simulink model "single_sat_attitude"  (R2018a)
settings: Solver=ode1  StartTime=0.0  StopTime=10.0  FixedStep=1/100  RelTol=1e-3
undefined symbols (not defined in the file or in its folder): Earth, h_init, hdmax, hmax, IAU, init, Kd, km, Kp, NRLMSISE_time_fromJD, q_init, s, wbn_init, WGS84
libraries: aerolibtransform2 x9, aerolibutil x6, sharedtransform x4, simulink x4, aerolibcelestial x3, vrlib x3, aerolibgravity2 x2, aerolibconvert2 x2, sharedutil x2, aerolibatmos2 x1
(part 1 of 2)
settings Model: Creator=nathan  LastModifiedBy=nathan
settings SolverCC: AutoInsertRateTranBlk=on

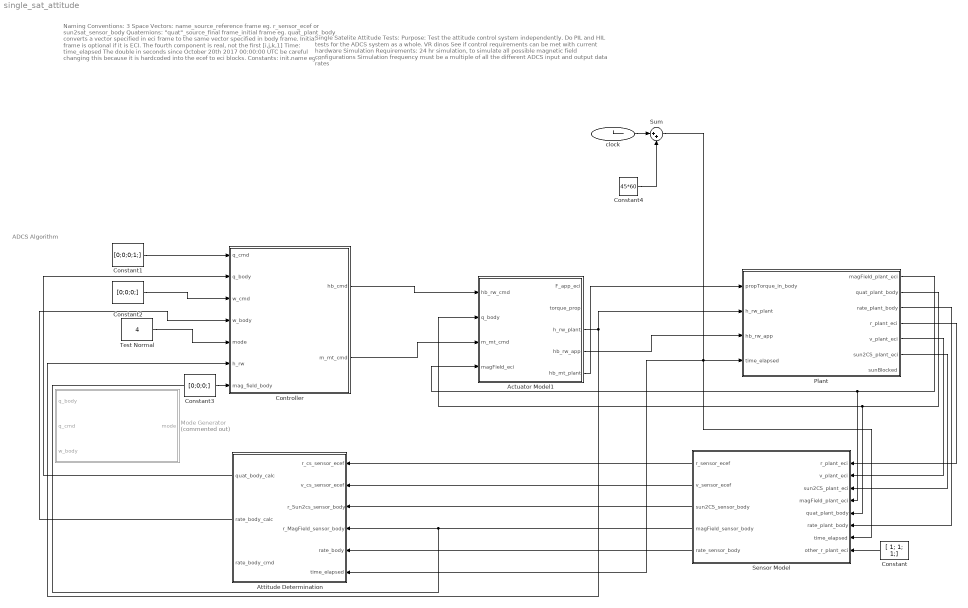
== system single_sat_attitude ==
  note: Naming Conventions:
      | 3 Space Vectors:
      | name_source_reference frame
      | eg. r_sensor_ecef or
      | sun2sat_sensor_body
      | Quaternions:
      | "quat"_source_final frame_initial frame
      | eg. quat_plant_body converts a vector specified in eci frame to the same vector specified in body frame.
      | Initial frame is optional if it is ECI.
      | The fourth component is real, not the first [i,j,k,1]
      | Time:
      | time_elapsed
      | The double in seconds since October 20th 2017 00:00:00 UTC
      | be careful changing this because it is hardcoded into the ecef to eci blocks.
      |
      | Constants:
      | init.name
      | eg. init.IMU0_MAG_RMS
      | Most constants that are not self explanitory should be stored in init. Their names must be all caps.
  note: ADCS Algorithm
  note: Single Satelite Attitude Tests:
      |
      | Purpose:
      | Test the attitude control system independently.
      | Do PIL and HIL tests for the ADCS system as a whole.
      | VR dinos
      | See if control requirements can be met with current hardware
      | Simulation Requirements:
      | 24 hr simulation, to simulate all possible magnetic field configurations
      | Simulation frequency must be a multiple of all the different ADCS input and output data rates
  Actuator Model1 : Subsystem
  Attitude Determination : Subsystem
  Constant : Constant  Value=[ 1; 1; 1;]
  Constant1 : Constant  Value=[0;0;0;1;]
  Constant2 : Constant  Value=[0;0;0;]
  Constant3 : Constant  Value=[0;0;0;]
  Constant4 : Constant  Value=45*60
  Controller : Subsystem
  Mode Generator : Stateflow chart  Commented=on  TreatAsAtomicUnit=on
  Plant : Subsystem
  Sensor Model : Subsystem
  Sum : Sum  Inputs=|++
  Test Normal : Constant  Value=4
  clock : Clock
      settings: Decimation=100
  wires:
  Actuator Model1/3(h_rw_plant) -> Plant/2(h_rw_plant), Controller/6(h_rw)
  Plant/3(rate_plant_body) -> Sensor Model/6(rate_plant_body)
  Plant/5(v_plant_eci) -> Sensor Model/2(v_plant_eci)
  Plant/4(r_plant_eci) -> Sensor Model/1(r_plant_eci)
  Plant/2(quat_plant_body) -> Actuator Model1/2(q_body), Sensor Model/5(quat_plant_body)
  Plant/1(magField_plant_eci) -> Actuator Model1/4(magField_eci), Sensor Model/4(magField_plant_eci)
  Controller/2(m_mt_cmd) -> Actuator Model1/3(m_mt_cmd)
  Controller/1(hb_cmd) -> Actuator Model1/1(hb_rw_cmd)
  Sensor Model/1(r_sensor_ecef) -> Attitude Determination/1(r_cs_sensor_ecef)
  Sensor Model/2(v_sensor_ecef) -> Attitude Determination/2(v_cs_sensor_ecef)
  Sensor Model/3(sun2CS_sensor_body) -> Attitude Determination/3(r_Sun2cs_sensor_body)
  Plant/6(sun2CS_plant_eci) -> Sensor Model/3(sun2CS_plant_eci)
  Constant/1 -> Sensor Model/8(other_r_plant_eci)
  Sensor Model/5(rate_sensor_body) -> Attitude Determination/5(rate_body)
  Sensor Model/4(magField_sensor_body) -> Controller/7(mag_field_body), Attitude Determination/4(r_MagField_sensor_body)
  Constant1/1 -> Controller/1(q_cmd)
  Constant2/1 -> Controller/3(w_cmd)
  Attitude Determination/2(rate_body_calc) -> Controller/4(w_body)
  Attitude Determination/1(quat_body_calc) -> Controller/2(q_body)
  Test Normal/1 -> Controller/5(mode)
  Constant3/1 -> ?
  clock/1 -> Sum/1
  Sum/1 -> Attitude Determination/6(time_elapsed), Sensor Model/7(time_elapsed), Plant/4(time_elapsed)
  Constant4/1 -> Sum/2
  Actuator Model1/4(hb_rw_app) -> Plant/3(hb_rw_app)
  Actuator Model1/5(hb_mt_plant) -> Plant/1("propTorque_in_body ")

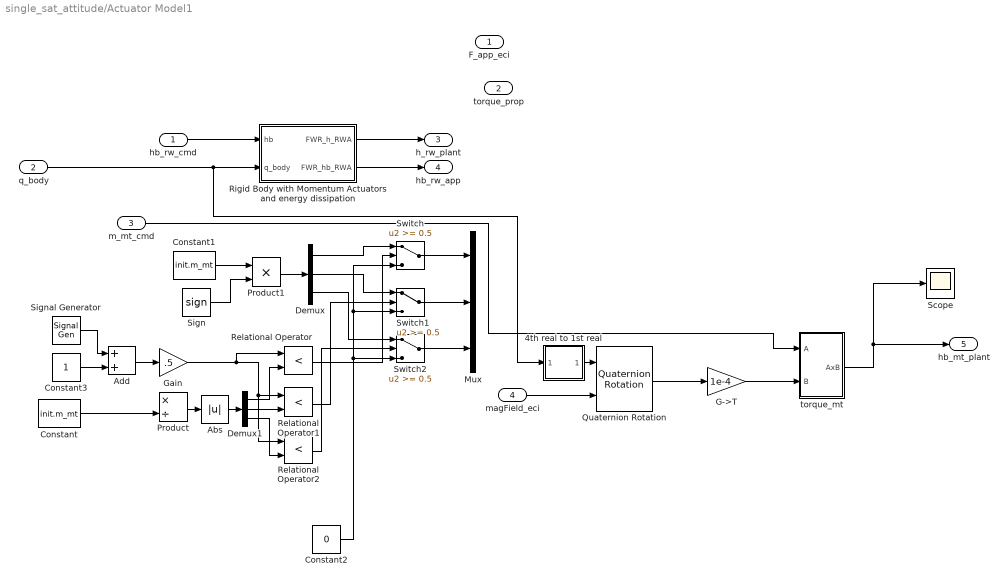
== system single_sat_attitude/Actuator Model1 ==
  hb_rw_cmd : Inport
  q_body : Inport  Port=2
  m_mt_cmd : Inport  Port=3
  magField_eci : Inport  Port=4  Unit=G  PortDimensions=3
  4th real to 1st real : Subsystem
  Abs : Abs  SaturateOnIntegerOverflow=on
  Add : Sum
  Constant : Constant  Value=init.m_mt
  Constant1 : Constant  Value=init.m_mt
  Constant2 : Constant  Value=0
  Constant3 : Constant
  Demux : Demux  Outputs=3
  Demux1 : Demux  Outputs=3
  G->T : Gain  Gain=1e-4
  Gain : Gain  Gain=.5
  Mux : Mux  Inputs=3
  Product : Product  Inputs=*/
  Product1 : Product
  Quaternion Rotation : aerolibutil/Quaternion Rotation
  Relational Operator : RelationalOperator  Operator=<  OutDataTypeStr=boolean  RndMeth=Simplest
  Relational Operator1 : RelationalOperator  Operator=<  OutDataTypeStr=boolean  RndMeth=Simplest
  Relational Operator2 : RelationalOperator  Operator=<  OutDataTypeStr=boolean  RndMeth=Simplest
  Rigid Body with Momentum Actuators and energy dissipation : Subsystem
  Scope : Scope
  Sign : Signum
  Signal Generator : SignalGenerator  WaveForm=sawtooth  Frequency=.5
  Switch : Switch  Threshold=0.5  SaturateOnIntegerOverflow=on  InputSameDT=on
  Switch1 : Switch  Threshold=0.5  SaturateOnIntegerOverflow=on  InputSameDT=on
  Switch2 : Switch  Threshold=0.5  SaturateOnIntegerOverflow=on  InputSameDT=on
  torque_mt : Subsystem
  F_app_eci : Outport
  torque_prop : Outport  Port=2
  h_rw_plant : Outport  Port=3
  hb_rw_app : Outport  Port=4
  hb_mt_plant : Outport  Port=5
  wires:
  Rigid Body with Momentum Actuators and energy dissipation/1(FWR_h_RWA) -> h_rw_plant/1
  Rigid Body with Momentum Actuators and energy dissipation/2(FWR_hb_RWA) -> hb_rw_app/1
  hb_rw_cmd/1 -> Rigid Body with Momentum Actuators and energy dissipation/1(hb)
  q_body/1 -> 4th real to 1st real/1(qin), Rigid Body with Momentum Actuators and energy dissipation/2(q_body)
  G->T/1 -> torque_mt/2(B)
  torque_mt/1(AxB) -> hb_mt_plant/1, Scope/1
  Constant/1 -> Product/2
  Product/1 -> Abs/1
  Constant1/1 -> Product1/1
  Sign/1 -> Product1/2
  Product1/1 -> Demux/1
  Switch2/1 -> Mux/3
  Switch1/1 -> Mux/2
  Switch/1 -> Mux/1
  Demux/1 -> Switch/1
  Demux/2 -> Switch1/1
  Demux/3 -> Switch2/1
  Relational Operator/1 -> Switch/2
  Relational Operator1/1 -> Switch1/2
  Relational Operator2/1 -> Switch2/2
  Constant2/1 -> Switch/3, Switch1/3, Switch2/3
  Abs/1 -> Demux1/1
  Demux1/1 -> Relational Operator/2
  Demux1/2 -> Relational Operator1/2
  Demux1/3 -> Relational Operator2/2
  Signal Generator/1 -> Add/1
  Constant3/1 -> Add/2
  Add/1 -> Gain/1
  Gain/1 -> Relational Operator2/1, Relational Operator1/1, Relational Operator/1
  m_mt_cmd/1 -> torque_mt/1(A)
  4th real to 1st real/1(qout) -> Quaternion Rotation/1
  Quaternion Rotation/1 -> G->T/1
  magField_eci/1 -> Quaternion Rotation/2

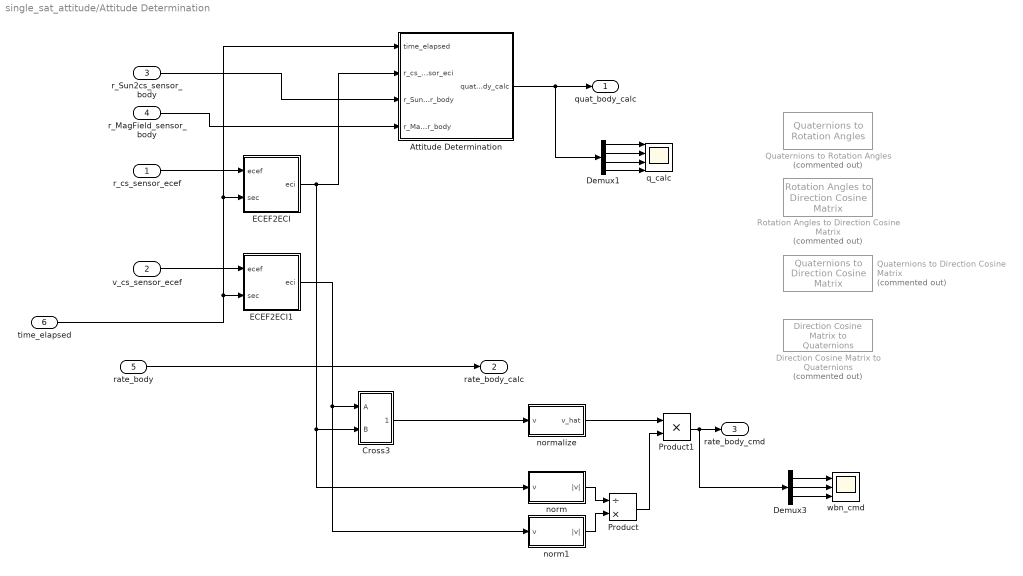
== system single_sat_attitude/Attitude Determination ==
  r_cs_sensor_ecef : Inport
  v_cs_sensor_ecef : Inport  Port=2
  r_Sun2cs_sensor_body : Inport  Port=3
  r_MagField_sensor_body : Inport  Port=4
  rate_body : Inport  Port=5
  time_elapsed : Inport  Port=6
  Attitude Determination : Subsystem
  Cross3 : Subsystem
  Demux1 : Demux
  Demux3 : Demux  Outputs=3
  Direction Cosine Matrix to Quaternions : sharedtransform/Direction Cosine Matrix  to Quaternions  Commented=on  aMode=aMode  action=None  tolerance=eps(2)
      settings: SourceProductName=Aerospace Blockset  SourceProductBaseCode=AE
  ECEF2ECI : Subsystem
  ECEF2ECI1 : Subsystem
  Product : Product  Inputs=/*
  Product1 : Product
  Quaternions to Direction Cosine Matrix : sharedtransform/Quaternions to  Direction Cosine Matrix  Commented=on  aMode=aMode
      settings: SourceProductName=Aerospace Blockset  SourceProductBaseCode=AE
  Quaternions to Rotation Angles : sharedtransform/Quaternions to Rotation Angles  Commented=on  rotationOrder=ZYX  aMode=aMode
      settings: SourceProductBaseCode=AE
  Rotation Angles to Direction Cosine Matrix : sharedtransform/Rotation Angles to Direction Cosine Matrix  Commented=on  rotationOrder=ZYX  aMode=aMode
      settings: SourceProductBaseCode=AE
  norm : Subsystem
  norm1 : Subsystem
  normalize : Subsystem
  q_calc : Scope  NumInputPorts=4
  wbn_cmd : Scope  NumInputPorts=3
  quat_body_calc : Outport
  rate_body_calc : Outport  Port=2
  rate_body_cmd : Outport  Port=3
  wires:
  rate_body/1 -> rate_body_calc/1
  time_elapsed/1 -> ECEF2ECI1/2(sec), ECEF2ECI/2(sec), Attitude Determination/1(time_elapsed)
  r_cs_sensor_ecef/1 -> ECEF2ECI/1(ecef)
  v_cs_sensor_ecef/1 -> ECEF2ECI1/1(ecef)
  ECEF2ECI/1(eci) -> norm/1(v), Cross3/2(B), Attitude Determination/2(r_cs_sensor_eci)
  ECEF2ECI1/1(eci) -> norm1/1(v), Cross3/1(A)
  r_Sun2cs_sensor_body/1 -> Attitude Determination/3(r_Sun2cs_sensor_body)
  r_MagField_sensor_body/1 -> Attitude Determination/4(r_MagField_sensor_body)
  Attitude Determination/1(quat_body_calc) -> Demux1/1, quat_body_calc/1
  Demux1/2 -> q_calc/2
  Demux1/1 -> q_calc/1
  Demux1/3 -> q_calc/3
  Demux1/4 -> q_calc/4
  Cross3/1(AxB) -> normalize/1(v)
  norm/1(|v|) -> Product/1
  norm1/1(|v|) -> Product/2
  Product/1 -> Product1/2
  normalize/1(v_hat) -> Product1/1
  Demux3/1 -> wbn_cmd/1
  Product1/1 -> Demux3/1, rate_body_cmd/1
  Demux3/3 -> wbn_cmd/3
  Demux3/2 -> wbn_cmd/2

== system single_sat_attitude/Controller ==
  note: 0- Power ON / Restart
      | 1- Detumble
      | 2- Regulation Control
      | 3- Tracking Control
      | 4- Thermal Safe
      | 5- Power Max
      | 6- Large Angle Slew
  note: 0- Power ON/restart
      | 1- Safe hold
      | 2- Detumble
      | 3- Large angle slew
      | 4- Normal
      | 5- Eclipse
      | 6- Docking
  q_cmd : Inport
  q_body : Inport  Port=2
  w_cmd : Inport  Port=3
  w_body : Inport  Port=4
  mode : Inport  Port=5
  h_rw : Inport  Port=6
  mag_field_body : Inport  Port=7
  Free Rigid Body with Momentum Actuators2 : Subsystem  Commented=on
  If : If  IfExpression=u1 == 0  ElseIfExpressions=u1 == 1, u1 == 2, u1 == 3, u1 == 4, u1==5
  Normal Mode Control System : Subsystem  TreatAsAtomicUnit=on
  hb_cmd : Outport
  m_mt_cmd : Outport  Port=2
  wires:
  q_cmd/1 -> Normal Mode Control System/1(q_cmd)
  q_body/1 -> Normal Mode Control System/2(q_body)
  w_cmd/1 -> Normal Mode Control System/3(w_cmd)
  w_body/1 -> Normal Mode Control System/4(w_body)
  mode/1 -> If/1
  If/5 -> Normal Mode Control System/Action
  Normal Mode Control System/1(hb_rw_cmd) -> hb_cmd/1
  mag_field_body/1 -> Normal Mode Control System/6(LDR_mag_field_body)
  Normal Mode Control System/2(m_mt_cmd) -> m_mt_cmd/1
  h_rw/1 -> Normal Mode Control System/5(LDR_h_rw)

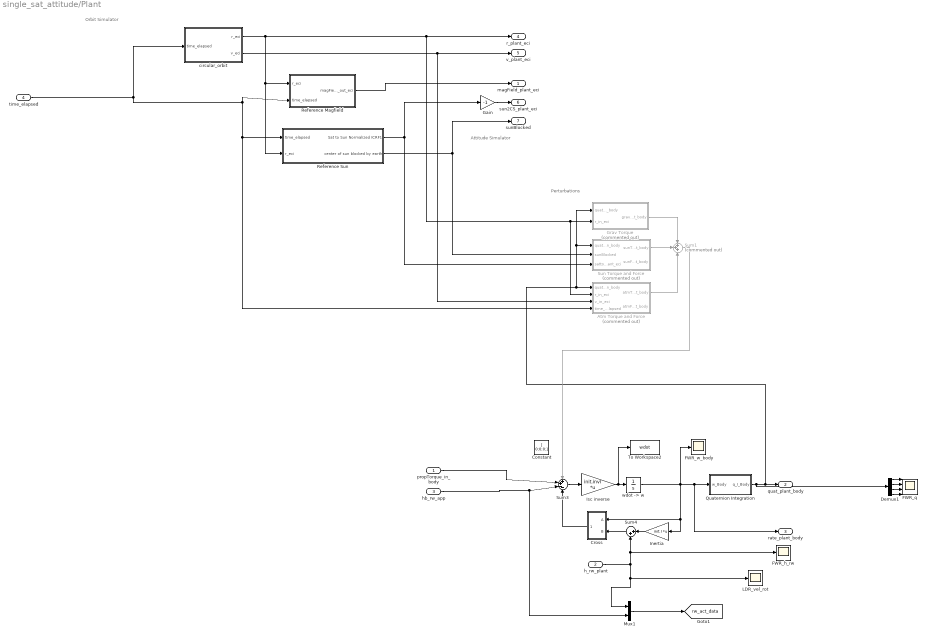
== system single_sat_attitude/Plant ==
  note: Perturbations
  note: Orbit Simulator
  note: Attitude Simulator
  "propTorque_in_body " : Inport
  h_rw_plant : Inport  Port=2
  hb_rw_app : Inport  Port=3
  time_elapsed : Inport  Port=4  Unit=s
  Atm Torque and Force : Subsystem  Commented=on  mask{Cd=init.Cd, areas=init.areas, unitnormals=init.unitnormals, comtocops=init.comtocops, jd=init.JD}
      mask prompts: Cd "Dimensionless drag coefficient. The drag coefficient is determined empirically, and is usually in the range between 1.5 and 2.5."; areas "Areas of the planes, units m^2. ([1, N]  vector)"; unitnormals "Normalzed unit vectors of planes. These point out of the plane into space. ([3, N]  vectors)"; comtocops "Vector distance from center of mass to center of pressure of each plane, units m. ([3, N]  vectors)"; jd "Inital Julian Date at time_elapsed=0."
      mask DialogControl DescGroupVar Prompt: Aerodynamic Torque and Force
      mask DialogControl DescTextVar Prompt: Outputs the torque and force in MKS in the body frame. The equations, parameters, and descriptions are from section 3.3.6.3 Aerodynamic Torque in Fundamentals of Spacecraft ADC. Uses the NRLMSISE-00 atmospheric model. Note this algorithm does not account for potential self-shielding that would exist on concave spacecraft.
  Constant : Constant  Value=[ 0;0;0;]
  Cross : Subsystem
  Demux1 : Demux
  "FWR_h_rw " : Scope
  FWR_q : Scope  NumInputPorts=4
  FWR_w_body : Scope
  Gain : Gain  Gain=-1
  Grav Torque : Subsystem  Commented=on  mask{inertia=init.I}
      mask prompts: inertia "Spacecraft inertia tensor, body frame."
      mask DialogControl DescGroupVar Prompt: Gravity Gradient Torque
      mask DialogControl DescTextVar Prompt: Outputs the torque and force in MKS in the body frame. The equations, parameters, and descriptions are from Table 10-18 in SMAD.
  Inertia : Gain  Gain=init.I  Multiplication=Matrix(K*u)  SaturateOnIntegerOverflow=on  OutDataTypeStr=Inherit: Same as input  ParamDataTypeStr=Inherit: Same as input
  Isc inverse : Gain  Gain=init.invI  Multiplication=Matrix(K*u)  SaturateOnIntegerOverflow=on  OutDataTypeStr=Inherit: Same as input  ParamDataTypeStr=Inherit: Same as input
  LDR_vel_rot : Scope
  Mux1 : Mux  Inputs=2
  Quaternion Integration : Subsystem
  "Reference Magfield " : Subsystem
  "Reference Sun " : Subsystem  mask{JD=init.JD}
      mask prompts: JD "Inital Julian Date at time_elapsed=0."
      mask DialogControl DescTextVar Prompt: Sun Reference, outputs the normalized vector from the input position to the sun in ICRF1 and using the DE405 effemeres model. For eclipse, the earth is assumed to be a sphere of radius 6371.0 km.
  Sum1 : Sum  Commented=on  Inputs=+++
  Sum3 : Sum  Inputs=++--  SaturateOnIntegerOverflow=on  InputSameDT=on  OutDataTypeStr=Inherit: Same as first input
  Sum4 : Sum  Inputs=|++
  Sun Torque and Force : Subsystem  Commented=on  mask{areas=init.areas, unitnormals=init.unitnormals, comtocops=init.comtocops, rss=init.rss, rds=init.rds}
      mask prompts: areas "Areas of the planes, units m^2. ([1, N]  vector)"; unitnormals "Normalzed unit vectors of planes. These point out of the plane into space. ([3, N]  vectors)"; comtocops "Vector distance from center of mass to center of pressure of each plane, units m. ([3, N]  vectors)"; rss "Surface specular reflectance coefficients. ([1, N]  vector)"; rds "Surface diffuse reflectance coefficients. ([1, N]  vector)"
      mask DialogControl DescGroupVar Prompt: Solar Radiation Torque and Force
      mask DialogControl DescTextVar Prompt: Outputs the torque and force in MKS in the body frame. The equations, parameters, and descriptions are from Table 10-18 in SMAD. Note this algorithm does not account for potential self-shielding that would exist on concave spacecraft.
  To Workspace2 : ToWorkspace  VariableName=wdot  SaveFormat=Timeseries  SampleTime=-1
  circular_orbit : Subsystem  mask{P=init.LDR.P, H=init.LDR.H}
      mask prompts: P "initial position in ECI, units m."; H "angular momuntum/mass in ECI units m^2/s"
      mask init:
      | W= norm(H)/dot(P,P); 
      | %angular rate magnitude, units rad/s
      | PPERP= cross(H,P)/norm(H); 
      | %position in orbit pi/2 phase shifted to the right from P, in ECI units m
      mask DialogControl DescTextVar Prompt: Circular Orbit Propagator
  "wdot -> w" : Integrator  InitialCondition=init.LDR.wbn
  magField_plant_eci : Outport  Unit=G  PortDimensions=3
  quat_plant_body : Outport  Port=2
  rate_plant_body : Outport  Port=3
  r_plant_eci : Outport  Port=4  Unit=m  PortDimensions=3
  v_plant_eci : Outport  Port=5  Unit=m/s  PortDimensions=3
  sun2CS_plant_eci : Outport  Port=6  PortDimensions=3
  sunBlocked : Outport  Port=7  OutDataTypeStr=boolean  PortDimensions=1
  tag scope: rw_act_data=global
  wires:
  "Reference Magfield "/1(magField_out_eci) -> magField_plant_eci/1
  Sum4/1 -> Cross/2(B)
  Isc inverse/1 -> To Workspace2/1, "wdot -> w"/1
  "wdot -> w"/1 -> Inertia/1, Cross/1(A), Quaternion Integration/1(w_Body), rate_plant_body/1, FWR_w_body/1
  Inertia/1 -> Sum4/1
  Quaternion Integration/1(q_I_Body) -> Grav Torque/1(quat_in_body), Sun Torque and Force/1(quat_in_body), Atm Torque and Force/1(quat_in_body), quat_plant_body/1, Demux1/1
  Demux1/2 -> FWR_q/2
  Demux1/1 -> FWR_q/1
  Demux1/3 -> FWR_q/3
  Demux1/4 -> FWR_q/4
  time_elapsed/1 -> "Reference Magfield "/2(time_elapsed), Atm Torque and Force/4(time_elapsed), "Reference Sun "/1(time_elapsed), circular_orbit/1(time_elapsed)
  circular_orbit/1(r_eci) -> r_plant_eci/1, Atm Torque and Force/2(r_in_eci), Grav Torque/2(r_in_eci), "Reference Sun "/2(r_eci), "Reference Magfield "/1(r_eci)
  circular_orbit/2(v_eci) -> v_plant_eci/1, Atm Torque and Force/3(v_in_eci)
  "Reference Sun "/2(center of sun blocked by earth) -> sunBlocked/1, Sun Torque and Force/2(sunBlocked)
  "Reference Sun "/1(Sat to Sun Normalized ICRF1) -> Gain/1, Sun Torque and Force/3(sattosun_plant_eci)
  Cross/1(AxB) -> Sum3/4
  "propTorque_in_body "/1 -> Sum3/2
  Grav Torque/1(gravT_out_body) -> Sum1/1
  Sun Torque and Force/1(sunT_out_body) -> Sum1/2
  Atm Torque and Force/1(atmT_out_body) -> Sum1/3
  Gain/1 -> sun2CS_plant_eci/1
  h_rw_plant/1 -> LDR_vel_rot/1, Mux1/1, "FWR_h_rw "/1, Sum4/2
  Mux1/1 -> [rw_act_data]
  hb_rw_app/1 -> Mux1/2, Sum3/3
  Sum3/1 -> Isc inverse/1
  Sum1/1 -> Sum3/1

== system single_sat_attitude/Sensor Model ==
  note: Gyroscope
  note: Magnetometer
  note: Sun Sensor
  r_plant_eci : Inport
  v_plant_eci : Inport  Port=2
  sun2CS_plant_eci : Inport  Port=3
  magField_plant_eci : Inport  Port=4  Unit=G
  quat_plant_body : Inport  Port=5
  rate_plant_body : Inport  Port=6
  time_elapsed : Inport  Port=7
  other_r_plant_eci : Inport  Port=8
  Data Type Conversion : DataTypeConversion  OutDataTypeStr=double
  Data Type Conversion1 : DataTypeConversion  Commented=through  OutDataTypeStr=double
  Data Type Conversion2 : DataTypeConversion  Commented=through  OutDataTypeStr=double
  Gyro : Subsystem  Commented=through
  Magnetometer : Subsystem  Commented=through
  Matrix Multiply2 : Product  Multiplication=Matrix(*)
  Matrix Multiply3 : Product  Multiplication=Matrix(*)
  Piksi GPS : Subsystem
  convert to m/s : Gain  Gain=1e-3
  convert to rad/s : Gain  Commented=through  Gain=1/init.IMU0_G_GN
  quat to DCM : Subsystem  mask(Direction Cosine Matrix){}
      mask help: Determines the 3x3 Direction Cosine Matrix (DCM) from a 4x1 quaternion orientation vector. The outputted DCM transforms vectors from inertial axes to body axes. This version corrects the fucked-up MATLAB one.
      mask Help:
      | <p>This block determines the 3x3 Direction Cosine Matrix (DCM) from a 4x1 quaternion orientation vector. The outputted DCM transforms vectors from inertial axes to body axes.  This version corrects the fucked-up MATLAB one</p>
      | 
      | <p>The block input and output contain more than one signal as described below.</p>
      | 
      | <p><H4>Block Vector Input - Quaternion</H4>
      | <ul>
      | <li>q0</li>
      | <li>q1</li>
      | <li>q2</li>
      | <li>q3</li>
      | </ul>
      | </p>
      | 
      | <p><H4>Block Matrix Output - Direction Cosine Matrix  </H4>
      |     <ul>
      |    </ul>
      |    </p>
      mask Display: disp('q to Q')
  r_sensor_ecef : Outport
  v_sensor_ecef : Outport  Port=2  Unit=m/s
  sun2CS_sensor_body : Outport  Port=3
  magField_sensor_body : Outport  Port=4  Unit=G
  rate_sensor_body : Outport  Port=5  Unit=rad/s
  wires:
  quat_plant_body/1 -> quat to DCM/1(e0 e1 e2 e3)
  sun2CS_plant_eci/1 -> Matrix Multiply3/2
  magField_plant_eci/1 -> Matrix Multiply2/2
  Matrix Multiply3/1 -> sun2CS_sensor_body/1
  quat to DCM/1(DCM) -> Matrix Multiply3/1, Matrix Multiply2/1
  r_plant_eci/1 -> Piksi GPS/2(r_plant_eci)
  v_plant_eci/1 -> Piksi GPS/4(v_plant_eci)
  time_elapsed/1 -> Piksi GPS/1(time_elapsed)
  Piksi GPS/4(pos_ecef) -> r_sensor_ecef/1
  Piksi GPS/6(vel_ecef) -> Data Type Conversion/1
  Matrix Multiply2/1 -> Magnetometer/1(Magnetic_Field_body)
  Magnetometer/1(Magxyz) -> Data Type Conversion1/1
  Gyro/1(sensor_w) -> Data Type Conversion2/1
  rate_plant_body/1 -> Gyro/1(body_w)
  other_r_plant_eci/1 -> Piksi GPS/3(other_r_plant_eci)
  Data Type Conversion/1 -> convert to m/s/1
  convert to m/s/1 -> v_sensor_ecef/1
  Data Type Conversion1/1 -> magField_sensor_body/1
  Data Type Conversion2/1 -> convert to rad/s/1
  convert to rad/s/1 -> rate_sensor_body/1

== system single_sat_attitude/Actuator Model1/4th real to 1st real ==
  qin : Inport
  Demux : Demux
  Mux : Mux
  qout : Outport
  wires:
  qin/1 -> Demux/1
  Demux/4 -> Mux/1
  Demux/1 -> Mux/2
  Demux/2 -> Mux/3
  Demux/3 -> Mux/4
  Mux/1 -> qout/1

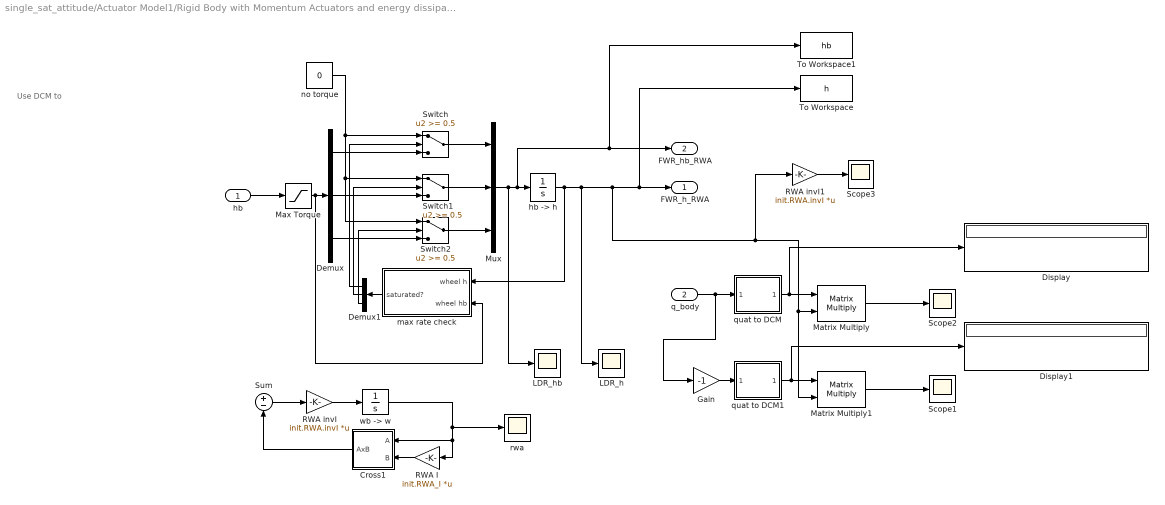
== system single_sat_attitude/Actuator Model1/Rigid Body with Momentum Actuators and energy dissipation ==
  note: Use DCM to
  hb : Inport
  q_body : Inport  Port=2
  Cross1 : Subsystem
  Demux : Demux  Outputs=3
  Demux1 : Demux  Outputs=3
  Display : Display
  Display1 : Display
  Gain : Gain  Gain=-1
  LDR_h : Scope
  LDR_hb : Scope
  Matrix Multiply : Product  Multiplication=Matrix(*)
  Matrix Multiply1 : Product  Multiplication=Matrix(*)
  Max Torque : Saturate  UpperLimit=init.hdmax  LowerLimit=-init.hdmax
  Mux : Mux  Inputs=3
  RWA I : Gain  Gain=init.RWA_I  Multiplication=Matrix(K*u)
  RWA invI : Gain  Gain=init.RWA.invI  Multiplication=Matrix(K*u)
  RWA invI1 : Gain  Gain=init.RWA.invI  Multiplication=Matrix(K*u)
  Scope1 : Scope
  Scope2 : Scope
  Scope3 : Scope
  Sum : Sum  Inputs=+|-
  Switch : Switch  Threshold=0.5  SaturateOnIntegerOverflow=on  InputSameDT=on
  Switch1 : Switch  Threshold=0.5  SaturateOnIntegerOverflow=on  InputSameDT=on
  Switch2 : Switch  Threshold=0.5  SaturateOnIntegerOverflow=on  InputSameDT=on
  To Workspace : ToWorkspace  VariableName=h  SaveFormat=Timeseries  SampleTime=-1
  To Workspace1 : ToWorkspace  VariableName=hb  SaveFormat=Timeseries  SampleTime=-1
  "hb -> h" : Integrator  InitialCondition=init.LDR.h
  max rate check : Subsystem
  no torque : Constant  Value=0
  quat to DCM : Subsystem  mask(Direction Cosine Matrix){}
      mask help: Determines the 3x3 Direction Cosine Matrix (DCM) from a 4x1 quaternion orientation vector. The outputted DCM transforms vectors from inertial axes to body axes. This version corrects the fucked-up MATLAB one.
      mask Help:
      | <p>This block determines the 3x3 Direction Cosine Matrix (DCM) from a 4x1 quaternion orientation vector. The outputted DCM transforms vectors from inertial axes to body axes.  This version corrects the fucked-up MATLAB one</p>
      | 
      | <p>The block input and output contain more than one signal as described below.</p>
      | 
      | <p><H4>Block Vector Input - Quaternion</H4>
      | <ul>
      | <li>q0</li>
      | <li>q1</li>
      | <li>q2</li>
      | <li>q3</li>
      | </ul>
      | </p>
      | 
      | <p><H4>Block Matrix Output - Direction Cosine Matrix  </H4>
      |     <ul>
      |    </ul>
      |    </p>
      mask Display: disp('q to Q')
  quat to DCM1 : Subsystem  mask(Direction Cosine Matrix){}
      mask help: Determines the 3x3 Direction Cosine Matrix (DCM) from a 4x1 quaternion orientation vector. The outputted DCM transforms vectors from inertial axes to body axes. This version corrects the fucked-up MATLAB one.
      mask Help:
      | <p>This block determines the 3x3 Direction Cosine Matrix (DCM) from a 4x1 quaternion orientation vector. The outputted DCM transforms vectors from inertial axes to body axes.  This version corrects the fucked-up MATLAB one</p>
      | 
      | <p>The block input and output contain more than one signal as described below.</p>
      | 
      | <p><H4>Block Vector Input - Quaternion</H4>
      | <ul>
      | <li>q0</li>
      | <li>q1</li>
      | <li>q2</li>
      | <li>q3</li>
      | </ul>
      | </p>
      | 
      | <p><H4>Block Matrix Output - Direction Cosine Matrix  </H4>
      |     <ul>
      |    </ul>
      |    </p>
      mask Display: disp('q to Q')
  rwa : Scope
  "wb -> w" : Integrator  InitialCondition=[0;0;0]
  FWR_h_RWA : Outport  PortDimensions=3
  FWR_hb_RWA : Outport  Port=2  PortDimensions=3
  wires:
  hb/1 -> Max Torque/1
  Mux/1 -> To Workspace1/1, FWR_hb_RWA/1, "hb -> h"/1, LDR_hb/1
  Max Torque/1 -> Demux/1, max rate check/2(wheel hb)
  max rate check/1(saturated?) -> Demux1/1
  Demux1/1 -> Switch/2
  Demux1/2 -> Switch1/2
  Demux1/3 -> Switch2/2
  no torque/1 -> Switch/1, Switch1/1, Switch2/1
  Demux/1 -> Switch/3
  Demux/2 -> Switch1/3
  Demux/3 -> Switch2/3
  Switch/1 -> Mux/1
  Switch1/1 -> Mux/2
  Switch2/1 -> Mux/3
  q_body/1 -> Gain/1, quat to DCM/1(e0 e1 e2 e3)
  quat to DCM/1(DCM) -> Display/1, Matrix Multiply/1
  Matrix Multiply/1 -> Scope2/1
  Matrix Multiply1/1 -> Scope1/1
  quat to DCM1/1(DCM) -> Display1/1, Matrix Multiply1/1
  "hb -> h"/1 -> max rate check/1(wheel h), RWA invI1/1, Matrix Multiply1/2, Matrix Multiply/2, To Workspace/1, FWR_h_RWA/1, LDR_h/1
  Gain/1 -> quat to DCM1/1(e0 e1 e2 e3)
  RWA I/1 -> Cross1/2(B)
  "wb -> w"/1 -> rwa/1, Cross1/1(A), RWA I/1
  Cross1/1(AxB) -> Sum/2
  Sum/1 -> RWA invI/1
  RWA invI/1 -> "wb -> w"/1
  RWA invI1/1 -> Scope3/1
  ? -> Sum/1

== system single_sat_attitude/Actuator Model1/torque_mt ==
  A : Inport
  B : Inport  Port=2
  Mux4 : Mux  Inputs=3
  Product{,1..5} (6 alike) : Product  SaturateOnIntegerOverflow=on  InputSameDT=on  OutDataTypeStr=Inherit: Same as first input
  Sum : Sum  Inputs=+-  SaturateOnIntegerOverflow=on  InputSameDT=on  OutDataTypeStr=Inherit: Same as first input
  Sum1 : Sum  Inputs=+-  SaturateOnIntegerOverflow=on  InputSameDT=on  OutDataTypeStr=Inherit: Same as first input
  Sum2 : Sum  Inputs=+-  SaturateOnIntegerOverflow=on  InputSameDT=on  OutDataTypeStr=Inherit: Same as first input
  demux2 : Demux  Outputs=3
  demux3 : Demux  Outputs=3
  AxB : Outport  InitialOutput=0
  wires:
  Mux4/1 -> AxB/1
  Sum2/1 -> Mux4/3
  Sum1/1 -> Mux4/2
  Sum/1 -> Mux4/1
  Product5/1 -> Sum2/2
  Product4/1 -> Sum2/1
  Product3/1 -> Sum1/2
  Product2/1 -> Sum1/1
  Product1/1 -> Sum/2
  Product/1 -> Sum/1
  demux3/1 -> Product5/2, Product2/2
  demux2/2 -> Product5/1, Product/1
  demux3/2 -> Product4/2, Product1/2
  demux2/1 -> Product4/1, Product3/1
  demux3/3 -> Product3/2, Product/2
  demux2/3 -> Product2/1, Product1/1
  B/1 -> demux3/1
  A/1 -> demux2/1

== system single_sat_attitude/Attitude Determination/Attitude Determination ==
  time_elapsed : Inport
  r_cs_sensor_eci : Inport  Port=2
  r_Sun2cs_sensor_body : Inport  Port=3
  r_MagField_sensor_body : Inport  Port=4
  Generate reference vectors from Ephemeris and Magnetic Field Model : Subsystem
  Subsystem : Subsystem
  quat_body_calc : Outport
  wires:
  r_cs_sensor_eci/1 -> Generate reference vectors from Ephemeris and Magnetic Field Model/2(r_cs_sensor_eci)
  time_elapsed/1 -> Generate reference vectors from Ephemeris and Magnetic Field Model/1(time_elapsed)
  r_Sun2cs_sensor_body/1 -> Subsystem/3(r_Sun2cs_sensor_body)
  r_MagField_sensor_body/1 -> Subsystem/4(r_MagField_sensor_body)
  Generate reference vectors from Ephemeris and Magnetic Field Model/1(r_Sun2cs_ref_eci) -> Subsystem/1(r_Sun2cs_ref_eci)
  Generate reference vectors from Ephemeris and Magnetic Field Model/2(r_MagField_ref_eci) -> Subsystem/2(r_MagField_ref_eci)
  Subsystem/1(quat_body_calc) -> quat_body_calc/1

== system single_sat_attitude/Attitude Determination/Cross3 ==
  A : Inport
  B : Inport  Port=2
  Mux4 : Mux  Inputs=3
  Product{,1..5} (6 alike) : Product  SaturateOnIntegerOverflow=on  InputSameDT=on  OutDataTypeStr=Inherit: Same as first input
  Sum : Sum  Inputs=+-  SaturateOnIntegerOverflow=on  InputSameDT=on  OutDataTypeStr=Inherit: Same as first input
  Sum1 : Sum  Inputs=+-  SaturateOnIntegerOverflow=on  InputSameDT=on  OutDataTypeStr=Inherit: Same as first input
  Sum2 : Sum  Inputs=+-  SaturateOnIntegerOverflow=on  InputSameDT=on  OutDataTypeStr=Inherit: Same as first input
  demux2 : Demux  Outputs=3
  demux3 : Demux  Outputs=3
  AxB : Outport  InitialOutput=0
  wires:
  A/1 -> demux2/1
  B/1 -> demux3/1
  demux2/3 -> Product1/1, Product2/1
  demux3/3 -> Product/2, Product3/2
  demux2/1 -> Product3/1, Product4/1
  demux3/2 -> Product1/2, Product4/2
  demux2/2 -> Product/1, Product5/1
  demux3/1 -> Product2/2, Product5/2
  Product/1 -> Sum/1
  Product1/1 -> Sum/2
  Product2/1 -> Sum1/1
  Product3/1 -> Sum1/2
  Product4/1 -> Sum2/1
  Product5/1 -> Sum2/2
  Sum/1 -> Mux4/1
  Sum1/1 -> Mux4/2
  Sum2/1 -> Mux4/3
  Mux4/1 -> AxB/1

== system single_sat_attitude/Attitude Determination/ECEF2ECI ==
  ecef : Inport
  sec : Inport  Port=2
  Direction Cosine Matrix ECI to ECEF : aerolibtransform2/Direction Cosine Matrix ECI to ECEF  red=IAU-2000/2006  year=init.year  month=October  day=20  hour=init.hour  min=init.min  sec=init.sec  deltaT=Sec  errorflag=Error  extraparamflag=off
      settings: AttributesFormatString=%<red>  SourceProductName=Aerospace Blockset  SourceProductBaseCode=AE
  Invert 3x3 Matrix : aerolibutil/Invert  3x3 Matrix
  Product1 : Product  Multiplication=Matrix(*)
  eci : Outport
  wires:
  Direction Cosine Matrix ECI to ECEF/1 -> Invert 3x3 Matrix/1
  Product1/1 -> eci/1
  sec/1 -> Direction Cosine Matrix ECI to ECEF/1
  Invert 3x3 Matrix/1 -> Product1/1
  ecef/1 -> Product1/2

== system single_sat_attitude/Attitude Determination/ECEF2ECI1 ==
  ecef : Inport
  sec : Inport  Port=2
  Direction Cosine Matrix ECI to ECEF : aerolibtransform2/Direction Cosine Matrix ECI to ECEF  red=IAU-2000/2006  year=init.year  month=October  day=20  hour=init.hour  min=init.min  sec=init.sec  deltaT=Sec  errorflag=Error  extraparamflag=off
      settings: AttributesFormatString=%<red>  SourceProductName=Aerospace Blockset  SourceProductBaseCode=AE
  Invert 3x3 Matrix : aerolibutil/Invert  3x3 Matrix
  Product1 : Product  Multiplication=Matrix(*)
  eci : Outport
  wires:
  Direction Cosine Matrix ECI to ECEF/1 -> Invert 3x3 Matrix/1
  Product1/1 -> eci/1
  sec/1 -> Direction Cosine Matrix ECI to ECEF/1
  ecef/1 -> Product1/2
  Invert 3x3 Matrix/1 -> Product1/1

== system single_sat_attitude/Attitude Determination/norm ==
  v : Inport
  Dot Product : DotProduct  InputSameDT=on  OutDataTypeStr=Inherit: Inherit via internal rule
  Math Function : Math  Operator=sqrt  SaturateOnIntegerOverflow=on
  |v| : Outport
  wires:
  Math Function/1 -> |v|/1
  Dot Product/1 -> Math Function/1
  v/1 -> Dot Product/2, Dot Product/1

== system single_sat_attitude/Attitude Determination/norm1 ==
  v : Inport
  Dot Product : DotProduct  InputSameDT=on  OutDataTypeStr=Inherit: Inherit via internal rule
  Math Function : Math  Operator=sqrt  SaturateOnIntegerOverflow=on
  |v| : Outport
  wires:
  v/1 -> Dot Product/1, Dot Product/2
  Dot Product/1 -> Math Function/1
  Math Function/1 -> |v|/1

== system single_sat_attitude/Attitude Determination/normalize ==
  v : Inport
  Dot Product : DotProduct  InputSameDT=on  OutDataTypeStr=Inherit: Inherit via internal rule
  Math Function : Math  Operator=sqrt  SaturateOnIntegerOverflow=on
  Product : Product  Inputs=*/  SaturateOnIntegerOverflow=on  InputSameDT=on  OutDataTypeStr=Inherit: Same as first input
  v_hat : Outport
  wires:
  v/1 -> Dot Product/1, Dot Product/2, Product/1
  Dot Product/1 -> Math Function/1
  Math Function/1 -> Product/2
  Product/1 -> v_hat/1

== system single_sat_attitude/Controller/Free Rigid Body with Momentum Actuators2 ==
  q_ref : Inport
  w_ref : Inport  Port=2
  "torque_pert " : Inport  Port=3
  Cross : Subsystem
  Demux1 : Demux
  Derivative Gain : Gain  Gain=Kd  SaturateOnIntegerOverflow=on  OutDataTypeStr=Inherit: Same as input  ParamDataTypeStr=Inherit: Same as input
  Inertia : Gain  Gain=init.I  Multiplication=Matrix(K*u)  SaturateOnIntegerOverflow=on  OutDataTypeStr=Inherit: Same as input  ParamDataTypeStr=Inherit: Same as input
  Isc inverse : Gain  Gain=init.invI  Multiplication=Matrix(K*u)  SaturateOnIntegerOverflow=on  OutDataTypeStr=Inherit: Same as input  ParamDataTypeStr=Inherit: Same as input
  Proportional Gain : Gain  Gain=Kp  SaturateOnIntegerOverflow=on  OutDataTypeStr=Inherit: Same as input  ParamDataTypeStr=Inherit: Same as input
  Quaternion Integration : Subsystem
  RWA Saturation Model (Maxon EC 32 Flat 15W 24V) : Subsystem
  Selector q(1:3) only1 : Selector  InputPortWidth=4  IndexOptions=Index vector (dialog)  Indices=[1 2 3]  OutputSizes=1
  Sum : Sum  Inputs=+--  SaturateOnIntegerOverflow=on  InputSameDT=on  OutDataTypeStr=Inherit: Same as first input
  Sum1 : Sum  Inputs=++|
  Sum3 : Sum  Inputs=|++
  compute attitude error : Subsystem
  quat_err : Scope  NumInputPorts=4
  torque_act : Scope
  torque_cmd : Scope
  "vel_rot " : Scope
  w_error : Sum  Inputs=+-
  "wdot -> w" : Integrator  InitialCondition=wbn_init
  quat : Outport
  rate : Outport  Port=2
  wires:
  Sum/1 -> Isc inverse/1
  Isc inverse/1 -> "wdot -> w"/1
  Cross/1(AxB) -> Sum/3
  Quaternion Integration/1(q_I_Body) -> compute attitude error/1(quat), quat/1
  q_ref/1 -> compute attitude error/2(quat_cmd)
  Selector q(1:3) only1/1 -> Proportional Gain/1
  w_error/1 -> Derivative Gain/1
  w_ref/1 -> w_error/2
  "wdot -> w"/1 -> w_error/1, Inertia/1, Cross/1(A), Quaternion Integration/1(w_Body), rate/1
  Demux1/4 -> quat_err/4
  Demux1/1 -> quat_err/1
  compute attitude error/1(quat error) -> Demux1/1, Selector q(1:3) only1/1
  Demux1/2 -> quat_err/2
  Demux1/3 -> quat_err/3
  "torque_pert "/1 -> Sum/1
  Derivative Gain/1 -> Sum1/2
  Proportional Gain/1 -> Sum1/1
  Sum3/1 -> Cross/2(B)
  Inertia/1 -> Sum3/1
  RWA Saturation Model (Maxon EC 32 Flat 15W 24V)/2(h_act) -> "vel_rot "/1, Sum3/2
  Sum1/1 -> torque_cmd/1, RWA Saturation Model (Maxon EC 32 Flat 15W 24V)/1(hb_com)
  RWA Saturation Model (Maxon EC 32 Flat 15W 24V)/1(hb_act) -> Sum/2, torque_act/1

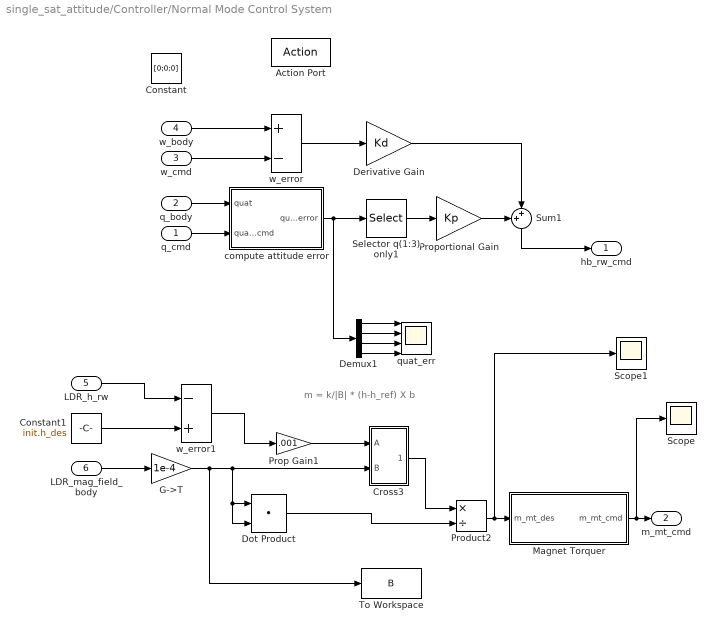
== system single_sat_attitude/Controller/Normal Mode Control System ==
  note: m = k/|B| * (h-h_ref) X b
  q_cmd : Inport
  q_body : Inport  Port=2
  w_cmd : Inport  Port=3
  w_body : Inport  Port=4
  LDR_h_rw : Inport  Port=5
  LDR_mag_field_body : Inport  Port=6
  Action Port : ActionPort  PropagateVarSize=During execution  ActionType=elseif
  Constant : Constant  Value=[0;0;0]
  Constant1 : Constant  Value=init.h_des
  Cross3 : Subsystem
  Demux1 : Demux
  Derivative Gain : Gain  Gain=Kd  SaturateOnIntegerOverflow=on  OutDataTypeStr=Inherit: Same as input  ParamDataTypeStr=Inherit: Same as input
  Dot Product : DotProduct  InputSameDT=on  OutDataTypeStr=Inherit: Inherit via internal rule
  G->T : Gain  Gain=1e-4
  Magnet Torquer : Subsystem
  Product2 : Product  Inputs=*/
  Prop Gain1 : Gain  Gain=.001
  Proportional Gain : Gain  Gain=Kp  SaturateOnIntegerOverflow=on  OutDataTypeStr=Inherit: Same as input  ParamDataTypeStr=Inherit: Same as input
  Scope : Scope
  Scope1 : Scope
  Selector q(1:3) only1 : Selector  InputPortWidth=4  IndexOptions=Index vector (dialog)  Indices=[1 2 3]  OutputSizes=1
  Sum1 : Sum  Inputs=++|
  To Workspace : ToWorkspace  VariableName=B  SaveFormat=Timeseries  SampleTime=-1
  compute attitude error : Subsystem
  quat_err : Scope  NumInputPorts=4
  w_error : Sum  Inputs=+-
  w_error1 : Sum  Inputs=-+
  hb_rw_cmd : Outport
  m_mt_cmd : Outport  Port=2
  wires:
  Proportional Gain/1 -> Sum1/1
  Derivative Gain/1 -> Sum1/2
  Demux1/2 -> quat_err/2
  w_error/1 -> Derivative Gain/1
  Demux1/3 -> quat_err/3
  Demux1/1 -> quat_err/1
  compute attitude error/1(quat error) -> Demux1/1, Selector q(1:3) only1/1
  w_body/1 -> w_error/1
  q_body/1 -> compute attitude error/1(quat)
  Demux1/4 -> quat_err/4
  q_cmd/1 -> compute attitude error/2(quat_cmd)
  Selector q(1:3) only1/1 -> Proportional Gain/1
  Sum1/1 -> hb_rw_cmd/1
  LDR_mag_field_body/1 -> G->T/1
  Dot Product/1 -> Product2/2
  Cross3/1(AxB) -> Product2/1
  Prop Gain1/1 -> Cross3/1(A)
  LDR_h_rw/1 -> w_error1/1
  w_error1/1 -> Prop Gain1/1
  Constant1/1 -> w_error1/2
  G->T/1 -> To Workspace/1, Dot Product/2, Dot Product/1, Cross3/2(B)
  w_cmd/1 -> w_error/2
  Product2/1 -> Scope1/1, Magnet Torquer/1(m_mt_des)
  Magnet Torquer/1(m_mt_cmd) -> Scope/1, m_mt_cmd/1

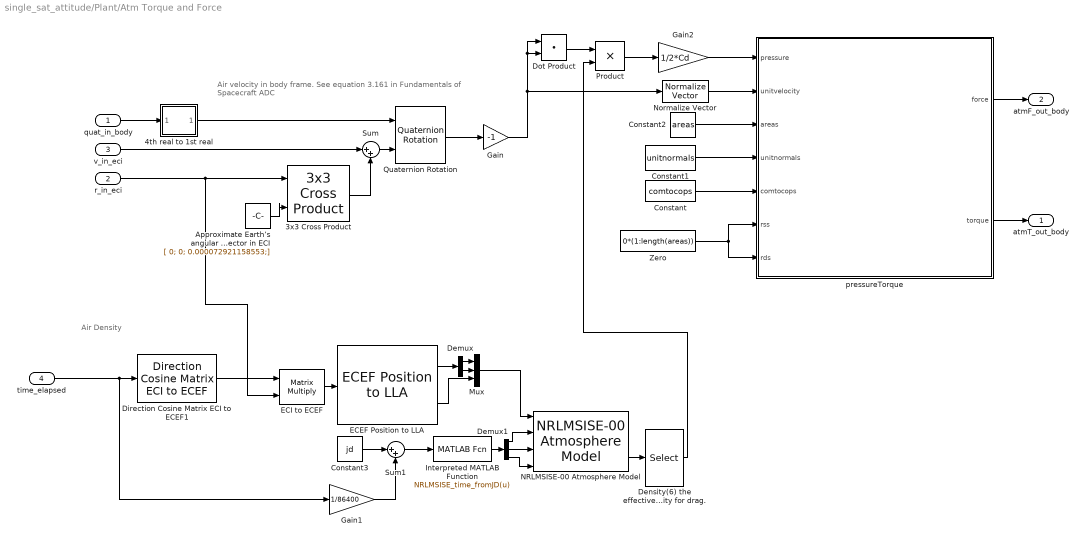
== system single_sat_attitude/Plant/Atm Torque and Force ==
  note: Air velocity in body frame.
      | See equation 3.161 in
      | Fundamentals of Spacecraft ADC
  note: Air Density
  quat_in_body : Inport  PortDimensions=4
  r_in_eci : Inport  Port=2  Unit=m  PortDimensions=3
  v_in_eci : Inport  Port=3  Unit=m/s  PortDimensions=3
  time_elapsed : Inport  Port=4  Unit=s  PortDimensions=1
  3x3 Cross Product : sharedutil/3x3 Cross Product  aMode=aMode
      settings: SourceProductBaseCode=AE
  4th real to 1st real : Subsystem
  Approximate Earth’s angular velocity vector in ECI : Constant  Value=[ 0; 0; 0.000072921158553;]
  Constant : Constant  Value=comtocops
  Constant1 : Constant  Value=unitnormals
  Constant2 : Constant  Value=areas
  Constant3 : Constant  Value=jd
  Demux : Demux  Outputs=2
  Demux1 : Demux  Outputs=3
  Density(6) the effective total mass density for drag. : Selector  InputPortWidth=9  IndexOptions=Index vector (dialog)  Indices=[6]  OutputSizes=1
  Direction Cosine Matrix ECI to ECEF1 : aerolibtransform2/Direction Cosine Matrix ECI to ECEF  red=IAU-2000/2006  year=init.year  month=October  day=20  hour=init.hour  min=init.min  sec=init.sec  deltaT=Sec  errorflag=Error  extraparamflag=off
      settings: AttributesFormatString=%<red>  SourceProductName=Aerospace Blockset  SourceProductBaseCode=AE
  Dot Product : DotProduct  InputSameDT=on  OutDataTypeStr=Inherit: Inherit via internal rule
  ECEF Position to LLA : aerolibtransform2/ECEF Position to LLA  units=Metric (MKS)  ptype=Earth (WGS84)  F=1/298.257223563  R=6378137
      settings: SourceProductName=Aerospace Blockset  SourceProductBaseCode=AE
  ECI to ECEF : Product  Multiplication=Matrix(*)  OutDataTypeStr=double
  Gain : Gain  Gain=-1
  Gain1 : Gain  Gain=1/86400
  Gain2 : Gain  Gain=1/2*Cd
  Interpreted MATLAB Function : MATLABFcn  MATLABFcn=NRLMSISE_time_fromJD(u)  OutputDimensions=3
  Mux : Mux  Inputs=3
  NRLMSISE-00 Atmosphere Model : aerolibatmos2/NRLMSISE-00 Atmosphere Model  units=Metric (MKS)  lst_input=off  flux_ap_input=off  flags_input=Internal  flags=ones(1,23)  oxygen_in=on  action=None
      settings: SourceProductName=Aerospace Blockset  SourceProductBaseCode=AE
  Normalize Vector : vrlib/Utilities/Normalize Vector  maxzero=0
      settings: SourceProductName=Simulink 3D Animation  SourceProductBaseCode=VR
  Product : Product
  Quaternion Rotation : aerolibutil/Quaternion Rotation
  Sum : Sum  Inputs=|++
  Sum1 : Sum  Inputs=|++
  Zero : Constant  Value=0*(1:length(areas))
  pressureTorque : MATLAB Function  TreatAsAtomicUnit=on
  atmT_out_body : Outport  Unit=N*m  PortDimensions=3
  atmF_out_body : Outport  Port=2  Unit=N  PortDimensions=3
  wires:
  pressureTorque/2(torque) -> atmT_out_body/1
  Zero/1 -> pressureTorque/7(rds), pressureTorque/6(rss)
  Constant/1 -> pressureTorque/5(comtocops)
  Constant1/1 -> pressureTorque/4(unitnormals)
  Constant2/1 -> pressureTorque/3(areas)
  Approximate Earth’s angular velocity vector in ECI/1 -> 3x3 Cross Product/2
  r_in_eci/1 -> 3x3 Cross Product/1, ECI to ECEF/2
  3x3 Cross Product/1 -> Sum/2
  v_in_eci/1 -> Sum/1
  Sum/1 -> Quaternion Rotation/2
  Normalize Vector/1 -> pressureTorque/2(unitvelocity)
  Quaternion Rotation/1 -> Gain/1
  Gain/1 -> Normalize Vector/1, Dot Product/1, Dot Product/2
  ECEF Position to LLA/1 -> Demux/1
  Demux/1 -> Mux/1
  Direction Cosine Matrix ECI to ECEF1/1 -> ECI to ECEF/1
  ECI to ECEF/1 -> ECEF Position to LLA/1
  ECEF Position to LLA/2 -> Mux/3
  Demux/2 -> Mux/2
  Mux/1 -> NRLMSISE-00 Atmosphere Model/1
  time_elapsed/1 -> Gain1/1, Direction Cosine Matrix ECI to ECEF1/1
  Gain1/1 -> Sum1/2
  Constant3/1 -> Sum1/1
  Sum1/1 -> Interpreted MATLAB Function/1
  Demux1/1 -> NRLMSISE-00 Atmosphere Model/2
  Demux1/2 -> NRLMSISE-00 Atmosphere Model/3
  Demux1/3 -> NRLMSISE-00 Atmosphere Model/4
  Dot Product/1 -> Product/1
  Product/1 -> Gain2/1
  Gain2/1 -> pressureTorque/1(pressure)
  pressureTorque/1(force) -> atmF_out_body/1
  4th real to 1st real/1(qout) -> Quaternion Rotation/1
  quat_in_body/1 -> 4th real to 1st real/1(qin)
  Interpreted MATLAB Function/1 -> Demux1/1
  NRLMSISE-00 Atmosphere Model/2 -> Density(6) the effective total mass density for drag./1
  Density(6) the effective total mass density for drag./1 -> Product/2

== system single_sat_attitude/Plant/Cross ==
  A : Inport
  B : Inport  Port=2
  Mux4 : Mux  Inputs=3
  Product{,1..5} (6 alike) : Product  SaturateOnIntegerOverflow=on  InputSameDT=on  OutDataTypeStr=Inherit: Same as first input
  Sum : Sum  Inputs=+-  SaturateOnIntegerOverflow=on  InputSameDT=on  OutDataTypeStr=Inherit: Same as first input
  Sum1 : Sum  Inputs=+-  SaturateOnIntegerOverflow=on  InputSameDT=on  OutDataTypeStr=Inherit: Same as first input
  Sum2 : Sum  Inputs=+-  SaturateOnIntegerOverflow=on  InputSameDT=on  OutDataTypeStr=Inherit: Same as first input
  demux2 : Demux  Outputs=3
  demux3 : Demux  Outputs=3
  AxB : Outport  InitialOutput=0
  wires:
  Mux4/1 -> AxB/1
  Sum2/1 -> Mux4/3
  Sum1/1 -> Mux4/2
  Sum/1 -> Mux4/1
  Product5/1 -> Sum2/2
  Product4/1 -> Sum2/1
  Product3/1 -> Sum1/2
  Product2/1 -> Sum1/1
  Product1/1 -> Sum/2
  Product/1 -> Sum/1
  demux3/1 -> Product5/2, Product2/2
  demux2/2 -> Product5/1, Product/1
  demux3/2 -> Product4/2, Product1/2
  demux2/1 -> Product4/1, Product3/1
  demux3/3 -> Product3/2, Product/2
  demux2/3 -> Product2/1, Product1/1
  B/1 -> demux3/1
  A/1 -> demux2/1

== system single_sat_attitude/Plant/Grav Torque ==
  quat_in_body : Inport  PortDimensions=4
  r_in_eci : Inport  Port=2  Unit=m  PortDimensions=3
  3x3 Cross Product : sharedutil/3x3 Cross Product  aMode=aMode
      settings: SourceProductBaseCode=AE
  3xEarth's gravitational coefficient : Gain  Gain=3*3.986E14
  4th real to 1st real : Subsystem
  Constant : Constant  Value=inertia
  Dot Product : DotProduct  InputSameDT=on  OutDataTypeStr=Inherit: Inherit via internal rule
  Fcn : Fcn  Expr=u^(-3)
  Gain : Gain  Gain=-1
  Multiply : Product  Multiplication=Matrix(*)
  Product : Product
  Quaternion Rotation : aerolibutil/Quaternion Rotation
  R0 : Sqrt  SaturateOnIntegerOverflow=on
  Unit vector toward nadir : vrlib/Utilities/Normalize Vector  maxzero=0
      settings: SourceProductName=Simulink 3D Animation  SourceProductBaseCode=VR
  gravT_out_body : Outport  Unit=N*m  PortDimensions=3
  wires:
  Dot Product/1 -> R0/1
  r_in_eci/1 -> Quaternion Rotation/2, Dot Product/2, Dot Product/1
  Quaternion Rotation/1 -> Gain/1
  Product/1 -> 3x3 Cross Product/1
  Constant/1 -> Multiply/1
  Gain/1 -> Unit vector toward nadir/1
  R0/1 -> Fcn/1
  Fcn/1 -> 3xEarth's gravitational coefficient/1
  3xEarth's gravitational coefficient/1 -> Product/1
  Unit vector toward nadir/1 -> Multiply/2, Product/2
  Multiply/1 -> 3x3 Cross Product/2
  3x3 Cross Product/1 -> gravT_out_body/1
  4th real to 1st real/1(qout) -> Quaternion Rotation/1
  quat_in_body/1 -> 4th real to 1st real/1(qin)

== system single_sat_attitude/Plant/Quaternion Integration ==
  w_Body : Inport
  Gain : Gain  Gain=-1
  Integrator1 : Integrator  InitialCondition=init.LDR.q_init  ContinuousStateAttributes='quaternion_plant'
  Selector : Selector  InputPortWidth=4  IndexOptions=Index vector (dialog)  Indices=4  OutputSizes=1
  Switch : Switch  Criteria=u2 > Threshold
  q_normalize : Subsystem
  qderiv : Subsystem
  q_I_Body : Outport
  wires:
  qderiv/1(qd) -> Integrator1/1
  Integrator1/1 -> q_normalize/1(q_in)
  q_normalize/1(q_out) -> Gain/1, Selector/1, q_I_Body/1, Switch/1, qderiv/2(q)
  w_Body/1 -> qderiv/1(w)
  Selector/1 -> Switch/2
  Gain/1 -> Switch/3

== system single_sat_attitude/Plant/Reference Magfield  ==
  r_eci : Inport  Unit=m  PortDimensions=3
  time_elapsed : Inport  Port=2  Unit=s  PortDimensions=1
  Constant1 : Constant  Value=init.decyear
  Demux : Demux  Commented=on  Outputs=2
  Direction Cosine Matrix ECEF to NED : aerolibtransform2/Direction Cosine Matrix ECEF to NED  Commented=on
      settings: SourceProductName=Aerospace Blockset  SourceProductBaseCode=AE
  Direction Cosine Matrix ECI to ECEF1 : aerolibtransform2/Direction Cosine Matrix ECI to ECEF  red=IAU-2000/2006  year=init.year  month=October  day=20  hour=init.hour  min=init.min  sec=init.sec  deltaT=Sec  errorflag=Error  extraparamflag=off
      settings: AttributesFormatString=%<red>  SourceProductName=Aerospace Blockset  SourceProductBaseCode=AE
  ECEF Position to LLA : aerolibtransform2/ECEF Position to LLA  Commented=on  units=Metric (MKS)  ptype=Earth (WGS84)  F=1/298.257223563  R=6378137
      settings: SourceProductName=Aerospace Blockset  SourceProductBaseCode=AE
  ECEF to ECI : Product  Multiplication=Matrix(*)  OutDataTypeStr=double
  ECI to ECEF : Product  Multiplication=Matrix(*)  OutDataTypeStr=double
  MATLAB Function : MATLAB Function  TreatAsAtomicUnit=on
  Product : Product  Commented=on  Multiplication=Matrix(*)
  Sum : Sum  Inputs=|++
  Transpose : Math  Commented=on  Operator=transpose  SaturateOnIntegerOverflow=on
  Transpose1 : Math  Operator=transpose  SaturateOnIntegerOverflow=on
  World Magnetic Model 2015 : aerolibgravity2/World Magnetic Model 2015  Commented=on  units=Metric (MKS)  time_in=on  month=January  day=1  year=2015  action=None  h_out=off  dec_out=off  inc_out=off  ti_out=off
      settings: SourceProductName=Aerospace Blockset  SourceProductBaseCode=AE
  nT_to_G : Gain  Commented=on  Gain=1e-5
  time elapsed to years : Gain  Gain=1/365/24/3600
  magField_out_eci : Outport  Unit=G  PortDimensions=3
  wires:
  ECEF Position to LLA/1 -> Demux/1, Direction Cosine Matrix ECEF to NED/1
  Direction Cosine Matrix ECEF to NED/1 -> Transpose/1
  Transpose/1 -> Product/1
  World Magnetic Model 2015/1 -> Product/2
  Product/1 -> nT_to_G/1
  Demux/1 -> World Magnetic Model 2015/2
  ECEF Position to LLA/2 -> World Magnetic Model 2015/1
  Sum/1 -> MATLAB Function/1(t), World Magnetic Model 2015/4
  Demux/2 -> World Magnetic Model 2015/3
  time elapsed to years/1 -> Sum/1
  Constant1/1 -> Sum/2
  time_elapsed/1 -> time elapsed to years/1, Direction Cosine Matrix ECI to ECEF1/1
  Direction Cosine Matrix ECI to ECEF1/1 -> Transpose1/1, ECI to ECEF/1
  r_eci/1 -> ECI to ECEF/2
  ECI to ECEF/1 -> MATLAB Function/2(x), ECEF Position to LLA/1
  Transpose1/1 -> ECEF to ECI/1
  ECEF to ECI/1 -> magField_out_eci/1
  MATLAB Function/1(B) -> ECEF to ECI/2

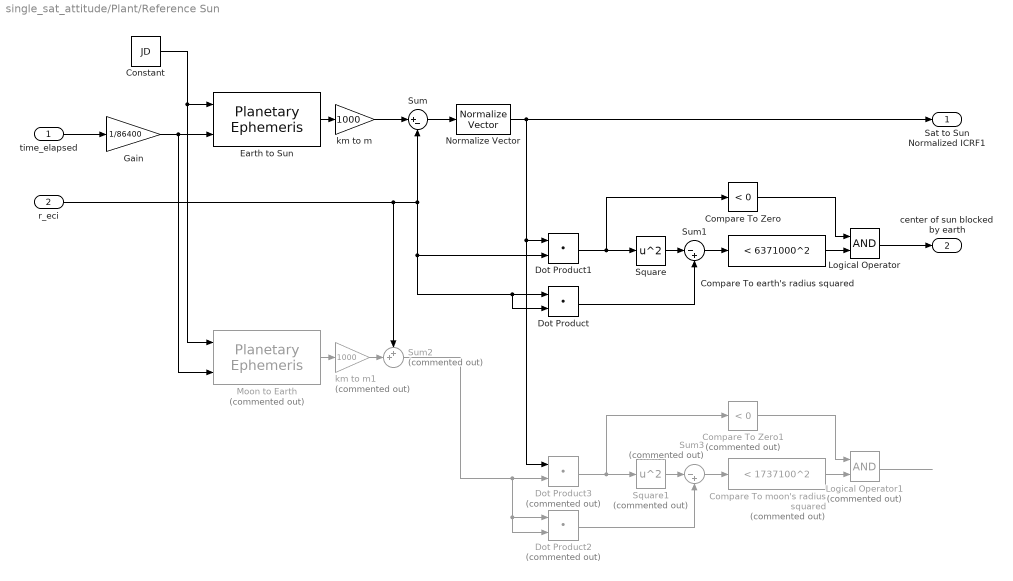
== system single_sat_attitude/Plant/Reference Sun  ==
  time_elapsed : Inport  Unit=s
  r_eci : Inport  Port=2  Unit=m  PortDimensions=3
  Compare To Zero : simulink/Logic and Bit Operations/Compare To Zero  relop=<  OutDataTypeStr=boolean
  Compare To Zero1 : simulink/Logic and Bit Operations/Compare To Zero  Commented=on  relop=<  OutDataTypeStr=boolean
  Compare To earth's radius squared : simulink/Logic and Bit Operations/Compare To Constant  relop=<  const=6371000^2  OutDataTypeStr=boolean
  Compare To moon's radius squared : simulink/Logic and Bit Operations/Compare To Constant  Commented=on  relop=<  const=1737100^2  OutDataTypeStr=boolean
  Constant : Constant  Value=JD
  Dot Product : DotProduct  InputSameDT=on  OutDataTypeStr=Inherit: Inherit via internal rule
  Dot Product1 : DotProduct  InputSameDT=on  OutDataTypeStr=Inherit: Inherit via internal rule
  Dot Product2 : DotProduct  Commented=on  InputSameDT=on  OutDataTypeStr=Inherit: Inherit via internal rule
  Dot Product3 : DotProduct  Commented=on  InputSameDT=on  OutDataTypeStr=Inherit: Inherit via internal rule
  Earth to Sun : aerolibcelestial/Planetary Ephemeris  kmflag=km,km/s  epochflag=T0 and elapsed Julian time  de=DE405  nCenter=Earth  nTarget=Sun  errorflag=Error  velflag=off
      settings: SourceProductName=Aerospace Blockset  SourceProductBaseCode=AE
  Gain : Gain  Gain=1/86400
  Logical Operator : Logic  AllPortsSameDT=off  OutDataTypeStr=boolean
  Logical Operator1 : Logic  Commented=on  AllPortsSameDT=off  OutDataTypeStr=boolean
  Moon to Earth : aerolibcelestial/Planetary Ephemeris  Commented=on  kmflag=km,km/s  epochflag=T0 and elapsed Julian time  de=DE405  nCenter=Moon  nTarget=Earth  errorflag=Error  velflag=off
      settings: SourceProductName=Aerospace Blockset  SourceProductBaseCode=AE
  Normalize Vector : vrlib/Utilities/Normalize Vector  maxzero=0
      settings: SourceProductName=Simulink 3D Animation  SourceProductBaseCode=VR
  Square : Math  Operator=square  SaturateOnIntegerOverflow=on
  Square1 : Math  Commented=on  Operator=square  SaturateOnIntegerOverflow=on
  Sum : Sum  Inputs=|+-
  Sum1 : Sum  Inputs=|-+
  Sum2 : Sum  Commented=on  Inputs=++|
  Sum3 : Sum  Commented=on  Inputs=|-+
  km to m : Gain  Gain=1000
  km to m1 : Gain  Commented=on  Gain=1000
  Sat to Sun Normalized ICRF1 : Outport  PortDimensions=3
  center of sun blocked by earth : Outport  Port=2  OutDataTypeStr=boolean  PortDimensions=1
  wires:
  time_elapsed/1 -> Gain/1
  Constant/1 -> Moon to Earth/1, Earth to Sun/1
  Gain/1 -> Moon to Earth/2, Earth to Sun/2
  Earth to Sun/1 -> km to m/1
  km to m/1 -> Sum/1
  Sum/1 -> Normalize Vector/1
  r_eci/1 -> Sum2/1, Dot Product1/2, Dot Product/2, Dot Product/1, Sum/2
  Dot Product1/1 -> Compare To Zero/1, Square/1
  Logical Operator/1 -> center of sun blocked by earth/1
  Sum1/1 -> Compare To earth's radius squared/1
  Compare To earth's radius squared/1 -> Logical Operator/2
  Compare To Zero/1 -> Logical Operator/1
  Square/1 -> Sum1/1
  Dot Product/1 -> Sum1/2
  Dot Product3/1 -> Compare To Zero1/1, Square1/1
  Compare To moon's radius squared/1 -> Logical Operator1/2
  Compare To Zero1/1 -> Logical Operator1/1
  Square1/1 -> Sum3/1
  Sum2/1 -> Dot Product2/1, Dot Product2/2, Dot Product3/2
  Logical Operator1/1 -> ?
  Dot Product2/1 -> Sum3/2
  Sum3/1 -> Compare To moon's radius squared/1
  Normalize Vector/1 -> Sat to Sun Normalized ICRF1/1, Dot Product3/1, Dot Product1/1
  Moon to Earth/1 -> km to m1/1
  km to m1/1 -> Sum2/2
